simulink library "NominalTrajectory"  (R2018b)
settings: Solver=VariableStepAuto  StartTime=0.0  StopTime=10.0  RelTol=1e-3
settings Model: Creator=BI28030  LastModifiedBy=BI28030

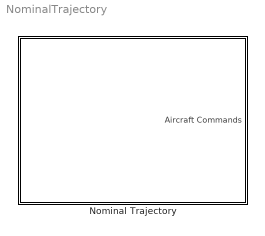
== system NominalTrajectory ==
  Nominal Trajectory : Subsystem  mask(Logic and Response: Nominal Trajectory){eventFilename=event1.mat, ts=.1}
      mask prompts: eventFilename "Event matrix mat filename"; ts "Dynamic Update Rate"
      mask help:
      | The "Nominal Trajectory" Logic and Response Block describes the nominal
      | trajectory of an aircraft as defined in a "event matrix" typically sampled
      | from the encounter model.
      |
      | Logic and Response: Nominal Trajectory loads aircaft motion
      | commands from a MATLAB MAT file containing an event matrix of climb rates,
      | turn rates, and longitudinal accelerations, and presents them as a
      | CASSATT v6 AircraftCommands bus.
      |
      | The specified MAT file must contain a single matrix variable with four
      | rows.  The rows are
      |   - Time of control value change in seconds
      |   - Climb rate in feet per second
      |   - Turn rate in radians per second
      |   - Longitudinal acceleration in feet per second squared
      |
      | These control quantities (climb rate, turn rate acceleration) are assumed
      | remain constant between the times specified in the event matrix (zero order
      | hold).  The first / last control values in the event matrix are assumed to
      | preexist / persist at the value infinitely backwards / forwards in time.
      mask init:
      | set_param( [ gcb '/FromFile' ], 'Filename', eventFilename )
      mask Help:
      | The "Nominal Trajectory" Logic and Response Block describes the nominal
      | trajectory of an aircraft as defined in a "event matrix" typically sampled
      | from the encounter model.
      | 
      | Logic and Response: Nominal Trajectory loads aircaft motion
      | commands from a MATLAB MAT file containing an event matrix of climb rates,
      | turn rates, and longitudinal accelerations, and presents them as a
      | CASSATT v6 AircraftCommands bus.
      | 
      | The specified MAT file must contain a single matrix variable with four
      | rows.  The rows are
      |   - Time of control value change in seconds
      |   - Climb rate in feet per second
      |   - Turn rate in radians per second
      |   - Longitudinal acceleration in feet per second squared
      | 
      | These control quantities (climb rate, turn rate acceleration) are assumed
      | remain constant between the times specified in the event matrix (zero order
      | hold).  The first / last control values in the event matrix are assumed to
      | preexist / persist at the value infinitely backwards / forwards in time.
      | 
      | CASSATT v6 Aircraft dynamics blocks, which calculate the positions and velocities
      | traced out by an aircraft's trajectory,
      | require input signals specifying controls for the aircraft (e.g. turn rate, acceleration, climb rate)
      | in the form of a AircraftCommands bus.
      | This block allows the user to specify what these controls in a Matlab MAT file.
      | Include this in your simulation to describe the nominal motion of an aircraft
      | trajectory you have sampled from the Lincoln Encounter Models.

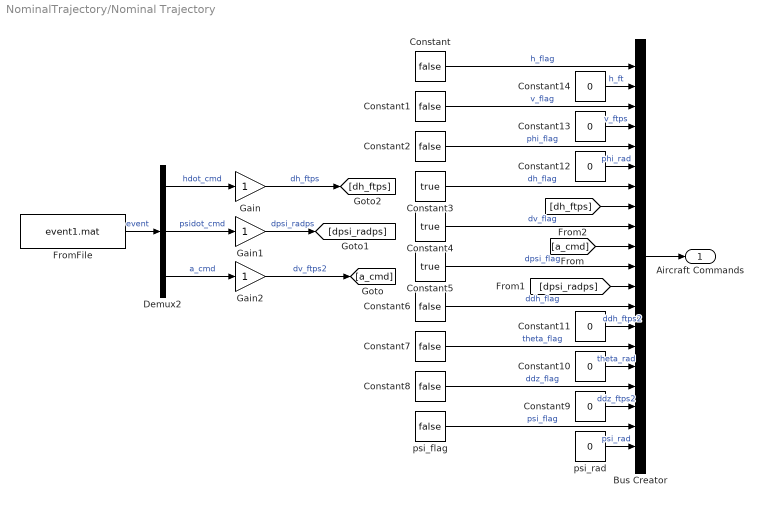
== system NominalTrajectory/Nominal Trajectory ==
  Bus Creator : BusCreator  Inputs=20  OutDataTypeStr=Bus: AircraftCommands  NonVirtualBus=on
  Constant{,1..2,6..8} (6 alike) : Constant  Value=false
  Constant{9..14} (6 alike) : Constant  Value=0
  Constant3 : Constant  Value=true
  Constant4 : Constant  Value=true
  Constant5 : Constant  Value=true
  Demux2 : Demux  Outputs=3
  FromFile : FromFile  FileName=event1.mat  SampleTime=ts  ExtrapolationBeforeFirstDataPoint=Hold first value  InterpolationWithinTimeRange=Zero order hold  ExtrapolationAfterLastDataPoint=Hold last value
  Gain : Gain
  Gain1 : Gain
  Gain2 : Gain
  psi_flag : Constant  Value=false
  psi_rad : Constant  Value=0
  Aircraft Commands : Outport  OutDataTypeStr=Bus: AircraftCommands
  wires:
  Constant12/1 -> Bus Creator/6  "phi_rad"
  Constant13/1 -> Bus Creator/4  "v_ftps"
  Constant14/1 -> Bus Creator/2  "h_ft"
  Constant10/1 -> Bus Creator/16  "theta_rad"
  Constant11/1 -> Bus Creator/14  "ddh_ftps2"
  Constant9/1 -> Bus Creator/18  "ddz_ftps2"
  Gain2/1 -> [a_cmd]  "dv_ftps2"
  Gain1/1 -> [dpsi_radps]  "dpsi_radps"
  Gain/1 -> [dh_ftps]  "dh_ftps"
  Constant8/1 -> Bus Creator/17  "ddz_flag"
  Constant7/1 -> Bus Creator/15  "theta_flag"
  Constant6/1 -> Bus Creator/13  "ddh_flag"
  Constant5/1 -> Bus Creator/11  "dpsi_flag"
  Constant4/1 -> Bus Creator/9  "dv_flag"
  Constant3/1 -> Bus Creator/7  "dh_flag"
  Constant2/1 -> Bus Creator/5  "phi_flag"
  Constant1/1 -> Bus Creator/3  "v_flag"
  Constant/1 -> Bus Creator/1  "h_flag"
  Bus Creator/1 -> Aircraft Commands/1
  FromFile/1 -> Demux2/1  "event"
  Demux2/3 -> Gain2/1  "a_cmd"
  Demux2/2 -> Gain1/1  "psidot_cmd"
  Demux2/1 -> Gain/1  "hdot_cmd"
  psi_flag/1 -> Bus Creator/19  "psi_flag"
  psi_rad/1 -> Bus Creator/20  "psi_rad"
  [a_cmd] -> Bus Creator/10
  [dpsi_radps] -> Bus Creator/12
  [dh_ftps] -> Bus Creator/8
